simulink model "End_Angle_verification"  (R2019b)
settings: Solver=VariableStepAuto  StartTime=0.0  StopTime=10.0  RelTol=1e-3
undefined symbols (not defined in the file): a
settings Model: Creator=zceeash  LastModifiedBy=arund
settings DebuggingCC: UnderSpecifiedDimensionMsg=warning

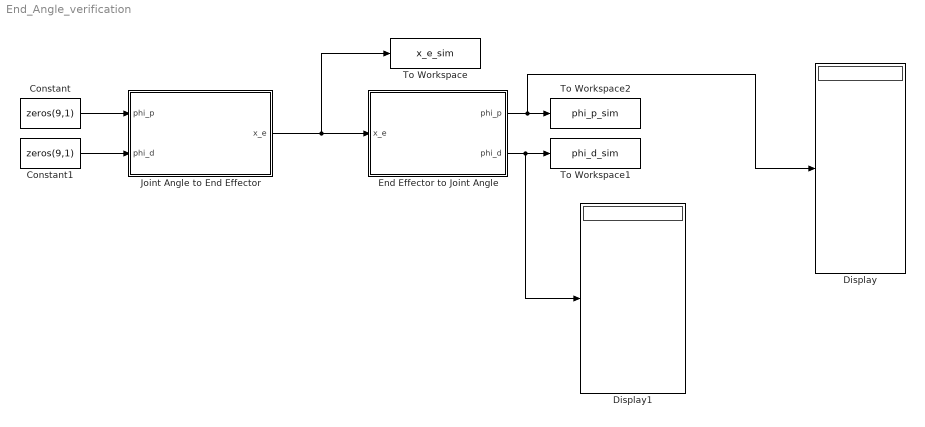
== system End_Angle_verification ==
  Constant : Constant  Value=zeros(9,1)
  Constant1 : Constant  Value=zeros(9,1)
  Display : Display
  Display1 : Display
  End Effector to Joint Angle : Subsystem
  Joint Angle to End Effector : Subsystem
  To Workspace : ToWorkspace  VariableName=x_e_sim  SaveFormat=Timeseries  SampleTime=-1
  To Workspace1 : ToWorkspace  VariableName=phi_d_sim  SaveFormat=Timeseries  SampleTime=-1
  To Workspace2 : ToWorkspace  VariableName=phi_p_sim  SaveFormat=Timeseries  SampleTime=-1
  wires:
  Joint Angle to End Effector/1(x_e) -> To Workspace/1, End Effector to Joint Angle/1(x_e)
  End Effector to Joint Angle/1(phi_p) -> Display/1, To Workspace2/1
  End Effector to Joint Angle/2(phi_d) -> Display1/1, To Workspace1/1
  Constant/1 -> Joint Angle to End Effector/1(phi_p)
  Constant1/1 -> Joint Angle to End Effector/2(phi_d)

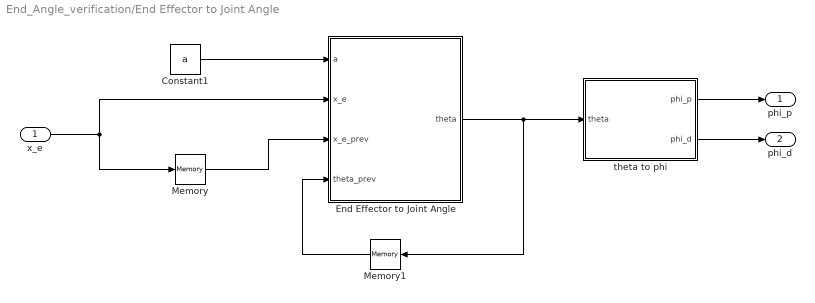
== system End_Angle_verification/End Effector to Joint Angle ==
  x_e : Inport
  Constant1 : Constant  Value=a
  "End Effector to Joint Angle " : MATLAB Function  TreatAsAtomicUnit=on
  Memory : Memory
  Memory1 : Memory
  theta to phi : MATLAB Function  TreatAsAtomicUnit=on
  phi_p : Outport
  phi_d : Outport  Port=2
  wires:
  x_e/1 -> Memory/1, "End Effector to Joint Angle "/2(x_e)
  Constant1/1 -> "End Effector to Joint Angle "/1(a)
  theta to phi/1(phi_p) -> phi_p/1
  theta to phi/2(phi_d) -> phi_d/1
  "End Effector to Joint Angle "/1(theta) -> theta to phi/1(theta), Memory1/1
  Memory1/1 -> "End Effector to Joint Angle "/4(theta_prev)
  Memory/1 -> "End Effector to Joint Angle "/3(x_e_prev)

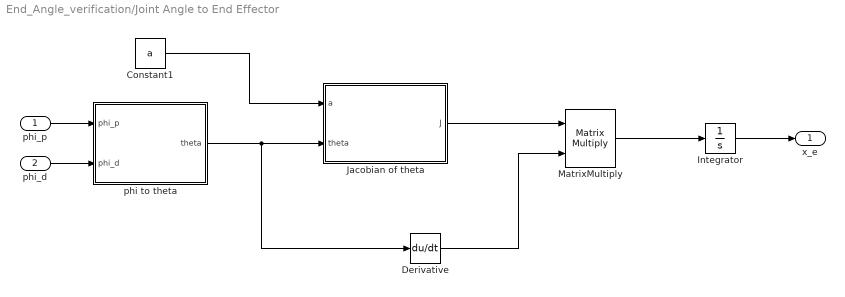
== system End_Angle_verification/Joint Angle to End Effector ==
  phi_p : Inport
  phi_d : Inport  Port=2
  Constant1 : Constant  Value=a
  Derivative : Derivative  CoefficientInTFapproximation=0
  Integrator : Integrator
  "Jacobian of theta " : MATLAB Function  TreatAsAtomicUnit=on
  MatrixMultiply : Product  Multiplication=Matrix(*)
  phi to theta : MATLAB Function  TreatAsAtomicUnit=on
  x_e : Outport
  wires:
  phi_p/1 -> phi to theta/1(phi_p)
  phi_d/1 -> phi to theta/2(phi_d)
  phi to theta/1(theta) -> "Jacobian of theta "/2(theta), Derivative/1
  "Jacobian of theta "/1(J) -> MatrixMultiply/1
  Derivative/1 -> MatrixMultiply/2
  MatrixMultiply/1 -> Integrator/1
  Integrator/1 -> x_e/1
  Constant1/1 -> "Jacobian of theta "/1(a)

== matlab function End_Angle_verification/Joint Angle to End Effector/Jacobian of theta  ==
  data: a input; J output; theta input
function J = fcn(a,theta)
N=9;
% Calculate D-H parameter table
DH_params=zeros(2*N,4);
for i=1:N
    if rem(i,2)==0
        DH_params(2*i-1:2*i,:)=[180+(theta(2*i-1)*180/pi) 90 0 0; 180+(theta(2*i)*180/pi) 0 a 0];
    else
        DH_params(2*i-1:2*i,:)=[(theta(2*i-1)*180/pi) 90 0 0; (theta(2*i)*180/pi) 0 a 0];
    end
end

% Calculate transformation matrix n_A_n+1 (A_wrt_prev) and store in cell
% array
A = cell(2*N,1);
for n=1:2*N
    theta_i=DH_params(n,1);
    alpha_i=DH_params(n,2);
    r_i=DH_params(n,3);
    d_i=DH_params(n,4);
    A{n}=[cosd(theta_i) -sind(theta_i)*cosd(alpha_i) sind(theta_i)*sind(alpha_i) r_i*cosd(theta_i);...
       sind(theta_i)  cosd(theta_i)*cosd(alpha_i) -cosd(theta_i)*sind(alpha_i) r_i*sind(theta_i);...
                  0              sind(alpha_i)   cosd(alpha_i)              d_i;...
                  0              0              0                         1];
end

% Create a list of transformation matrices wrt base for all joints
A_till_prev_wrt_base=cell(2*N,1);
A_till_prev_wrt_base{1}=eye(4);
for n=1:2*N-1
    A_till_prev_wrt_base{n+1}=A_till_prev_wrt_base{n}*A{n};
end
A_2N=A_till_prev_wrt_base{2*N}*A{2*N};
% Create Jacobian
J=zeros(6,2*N);
for n=1:2*N
    J_v=cross((A_till_prev_wrt_base{n}(1:3,1:3)*[0;0;1]),(A_2N(1:3,4)-A_till_prev_wrt_base{n}(1:3,4)));
    J_w=A_till_prev_wrt_base{n}(1:3,1:3)*[0;0;1];
    J(:,n)=[J_v;J_w];
end

== matlab function End_Angle_verification/End Effector to Joint Angle/End Effector to Joint Angle  ==
  data: a input; x_e input; x_e_prev input; theta output; theta_prev input
function theta  = fcn(a,x_e,x_e_prev,theta_prev)
N=9;
error_tol=1/1000;

theta=zeros(2*N,1);

theta_j=zeros(2*N,1);

%Numerical iteration to find solution
for j=0:10000
% Calculate x_e_j
% Calculate D-H parameter table
DH_params=zeros(2*N,4);
for i=1:N
    if rem(i,2)==0
        DH_params(2*i-1:2*i,:)=[180+(theta_j(2*i-1)*180/pi) 90 0 0; 180+(theta_j(2*i)*180/pi) 0 a 0];
    else
        DH_params(2*i-1:2*i,:)=[(theta_j(2*i-1)*180/pi) 90 0 0; (theta_j(2*i)*180/pi) 0 a 0];
    end
end

% Calculate transformation matrix n_A_n+1 (A_wrt_prev) and store in cell
% array
A = cell(2*N,1);
for n=1:2*N
    theta_i=DH_params(n,1);
    alpha_i=DH_params(n,2);
    r_i=DH_params(n,3);
    d_i=DH_params(n,4);
    A{n}=[cosd(theta_i) -sind(theta_i)*cosd(alpha_i) sind(theta_i)*sind(alpha_i) r_i*cosd(theta_i);...
       sind(theta_i)  cosd(theta_i)*cosd(alpha_i) -cosd(theta_i)*sind(alpha_i) r_i*sind(theta_i);...
                  0              sind(alpha_i)   cosd(alpha_i)              d_i;...
                  0              0              0                         1];
end

% Create a list of transformation matrices wrt base for all joints
A_till_prev_wrt_base=cell(2*N,1);
A_till_prev_wrt_base{1}=eye(4);
for n=1:2*N-1
    A_till_prev_wrt_base{n+1}=A_till_prev_wrt_base{n}*A{n};
end
A_2N=A_till_prev_wrt_base{2*N}*A{2*N};
% Create Jacobian
J=zeros(6,2*N);
for n=1:2*N
    J_v=cross((A_till_prev_wrt_base{n}(1:3,1:3)*[0;0;1]),(A_2N(1:3,4)-A_till_prev_wrt_base{n}(1:3,4)));
    J_w=A_till_prev_wrt_base{n}(1:3,1:3)*[0;0;1];
    J(:,n)=[J_v;J_w];
end

   x_e_j = J*(theta_j-theta_prev) + x_e_prev;
   % Get error
   x_e_j_error = x_e - x_e_j;
   if norm(x_e_j_error) <= (error_tol*N)
       theta = theta_j;
       break
   end
   % Use error to estimate delta_theta
   J_inv=pinv(J);
   delta_theta_j= J_inv*x_e_j_error;
   % Update theta_j
   theta_j = theta_j + delta_theta_j;
   
   if j==10000
       theta=ones(2*N,1)*NaN;
   end
end
if all(isnan(theta(:)))
    disp('Could not find solution!')
end
end

== matlab function End_Angle_verification/Joint Angle to End Effector/phi to theta ==
  data: phi_p input; theta output; phi_d input
function theta = fcn(phi_p,phi_d)
N=9;
% Create theta
theta=zeros(2*N,1);
for n=1:N
    theta(2*n-1:2*n)=[(-1)^(n+1)*phi_p(n);phi_d(n)];
end

== matlab function End_Angle_verification/End Effector to Joint Angle/theta to phi ==
  data: theta input; phi_p output; phi_d output
function [phi_p,phi_d] = fcn(theta)
N=9;
% Create theta
phi_p=theta(1:2:2*N-1);
for n=1:N
    phi_p(n)=(-1)^(n+1)*phi_p(n);
end
phi_d=theta(2:2:2*N);
